simulink model "Enceinte_climatique_original"  (R2024b)
settings: Solver=VariableStepAuto  StartTime=0.0  StopTime=6  RelTol=1e-3
settings Model: Creator=boiteth  LastModifiedBy=boiteth

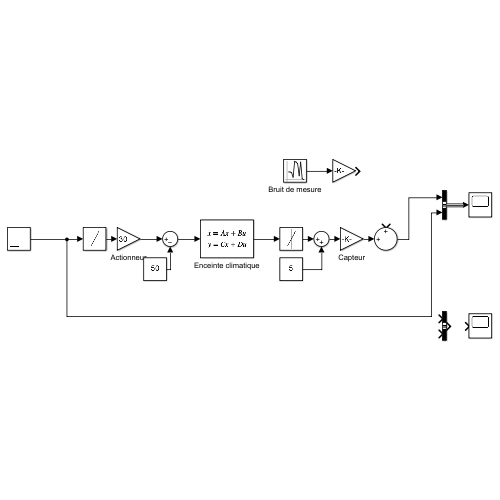
[thumbnail: Simulink's stored preview of the top-level diagram]
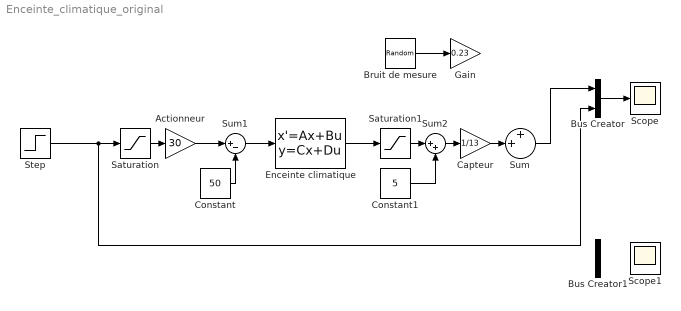
== system Enceinte_climatique_original ==
  Actionneur : Gain  Gain=30
  Bruit de mesure : RandomNumber  Variance=0.4  Seed=2  SampleTime=0.1
  Bus Creator : BusCreator  Inputs=2
  Bus Creator1 : BusCreator  Inputs=2
  Capteur : Gain  Gain=1/13
  Constant : Constant  Value=50
  Constant1 : Constant  Value=5
  Enceinte climatique : StateSpace  A=-2  B=2  D=0  InitialCondition=0
  Gain : Gain  Gain=0.23
  Saturation : Saturate  UpperLimit=5  LowerLimit=0
  Saturation1 : Saturate  UpperLimit=5  LowerLimit=0
  Scope : Scope
  Scope1 : Scope
  Step : Step  Before=1.15  After=2.7  SampleTime=0
  Sum : Sum  Inputs=++|
  Sum1 : Sum  Inputs=|+-
  Sum2 : Sum  Inputs=|++
  wires:
  Step/1 -> Bus Creator/2, Saturation/1
  Saturation/1 -> Actionneur/1
  Enceinte climatique/1 -> Saturation1/1
  Sum/1 -> Bus Creator/1
  Bus Creator/1 -> Scope/1
  Bruit de mesure/1 -> Gain/1
  Actionneur/1 -> Sum1/1
  Constant/1 -> Sum1/2
  Sum1/1 -> Enceinte climatique/1
  Capteur/1 -> Sum/2
  Saturation1/1 -> Sum2/1
  Sum2/1 -> Capteur/1
  Constant1/1 -> Sum2/2
